simulink model "task3_4"  (R2020b)
settings: Solver=FixedStepAuto  StartTime=0.0  StopTime=90.0  FixedStep=0.01  RelTol=1e-3
undefined symbols (not defined in the file or in its folder): alpha, DiscIntNeverNeededParam
settings Model: Creator=hauss  LastModifiedBy=hauss

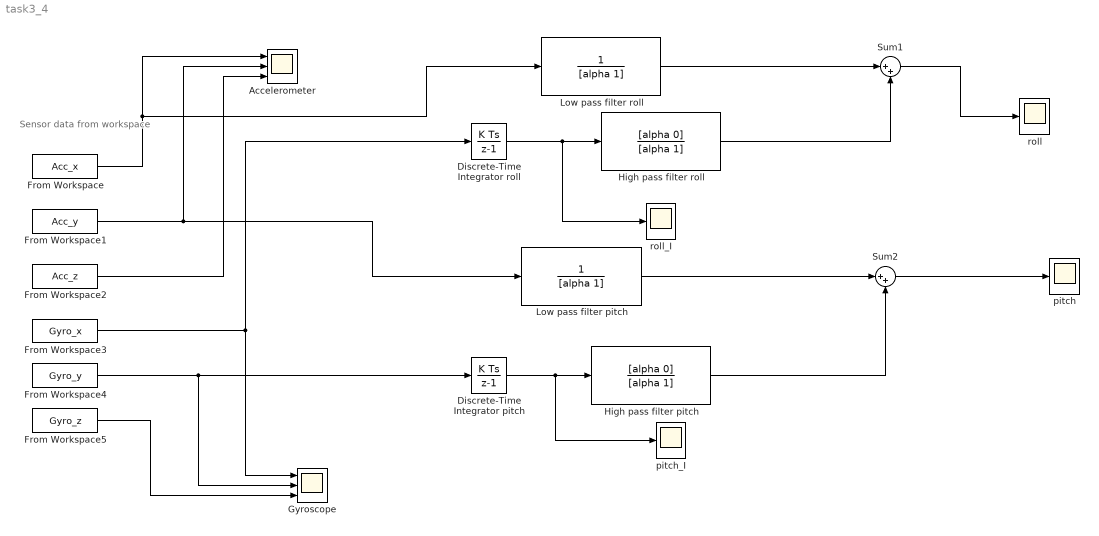
== system task3_4 ==
  note: Sensor data from
      | workspace
  Accelerometer : Scope  NumInputPorts=3
  Discrete-Time Integrator pitch : DiscreteIntegrator  SampleTime=-1  ICPrevOutput=DiscIntNeverNeededParam  ICPrevScaledInput=DiscIntNeverNeededParam
  Discrete-Time Integrator roll : DiscreteIntegrator  SampleTime=-1  ICPrevOutput=DiscIntNeverNeededParam  ICPrevScaledInput=DiscIntNeverNeededParam
  From Workspace : FromWorkspace  VariableName=Acc_x
  From Workspace1 : FromWorkspace  VariableName=Acc_y
  From Workspace2 : FromWorkspace  VariableName=Acc_z
  From Workspace3 : FromWorkspace  VariableName=Gyro_x
  From Workspace4 : FromWorkspace  VariableName=Gyro_y
  From Workspace5 : FromWorkspace  VariableName=Gyro_z
  Gyroscope : Scope  NumInputPorts=3
  High pass filter pitch : TransferFcn  Numerator=[alpha 0]  Denominator=[alpha 1]
  High pass filter roll : TransferFcn  Numerator=[alpha 0]  Denominator=[alpha 1]
  Low pass filter pitch : TransferFcn  Denominator=[alpha 1]
  Low pass filter roll : TransferFcn  Denominator=[alpha 1]
  Sum1 : Sum  Inputs=|++
  Sum2 : Sum  Inputs=|++
  pitch : Scope
  pitch_I : Scope
  roll : Scope
  roll_I : Scope
  wires:
  From Workspace/1 -> Low pass filter roll/1, Accelerometer/1
  From Workspace1/1 -> Accelerometer/2, Low pass filter pitch/1
  From Workspace2/1 -> Accelerometer/3
  From Workspace3/1 -> Discrete-Time Integrator roll/1, Gyroscope/1
  From Workspace4/1 -> Discrete-Time Integrator pitch/1, Gyroscope/2
  From Workspace5/1 -> Gyroscope/3
  High pass filter roll/1 -> Sum1/2
  Low pass filter roll/1 -> Sum1/1
  Discrete-Time Integrator roll/1 -> roll_I/1, High pass filter roll/1
  Sum1/1 -> roll/1
  Discrete-Time Integrator pitch/1 -> High pass filter pitch/1, pitch_I/1
  Low pass filter pitch/1 -> Sum2/1
  High pass filter pitch/1 -> Sum2/2
  Sum2/1 -> pitch/1
